simulink model "fly"  (Simulink 7.9)
settings: Solver=ode45  StartTime=0.0  StopTime=2  RelTol=1e-3
libraries: simulink x1
settings Model: Creator=tbourke  LastModifiedBy=tbourke

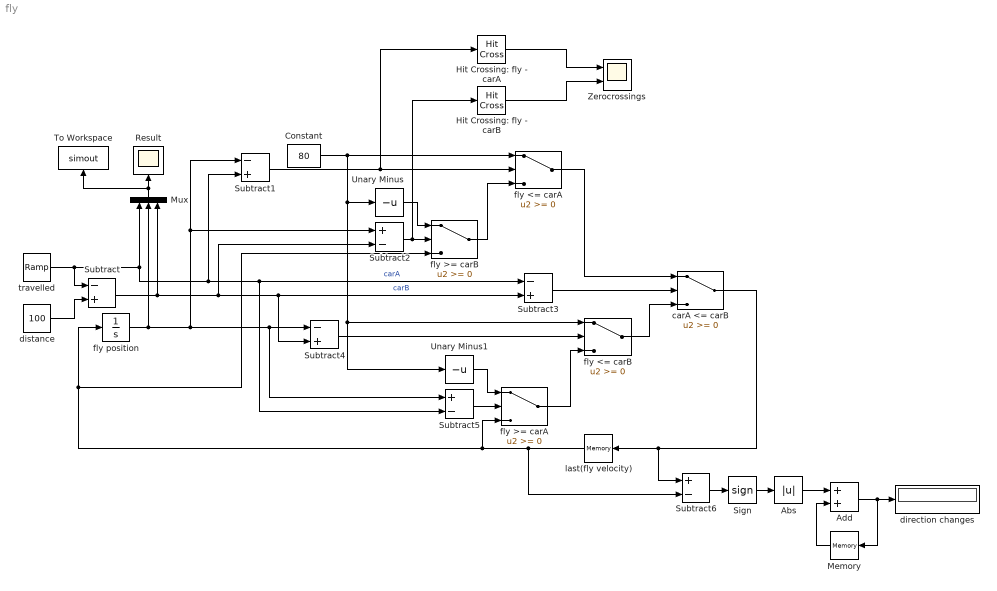
== system fly ==
  Abs : Abs
  Add : Sum
  Constant : Constant  Value=80
  Hit Crossing: fly - carA : HitCross
  Hit Crossing: fly - carB : HitCross
  Memory : Memory
  Mux : Mux  Inputs=3
  Result : Scope
      settings: TimeRange=2  YMin=0  YMax=100  SaveName=result  MaxDataPoints=500000  SampleInput=on
  Sign : Signum
  Subtract{,1,3..4} (4 alike) : Sum  Inputs=-+
  Subtract2 : Sum  Inputs=+-
  Subtract5 : Sum  Inputs=+-
  Subtract6 : Sum  Inputs=+-
  To Workspace : ToWorkspace  VariableName=simout  SampleTime=-1
  Unary Minus : UnaryMinus
  Unary Minus1 : UnaryMinus
  Zerocrossings : Scope  NumInputPorts=2
      settings: TimeRange=2  YMin=0~0  YMax=1~1  SaveName=zerocrossings  MaxDataPoints=500000  SampleInput=on
  carA <= carB : Switch
  direction changes : Display
  distance : Constant  Value=100
  fly <= carA : Switch
  fly <= carB : Switch
  fly >= carA : Switch
  fly >= carB : Switch
  fly position : Integrator
  last(fly velocity) : Memory  X0=80
  travelled : simulink/Sources/Ramp  slope=50  start=0  X0=0
  wires:
  Subtract3/1 -> carA <= carB/2
  distance/1 -> Subtract/2
  travelled/1 -> Subtract/1, Subtract1/2, Subtract3/1, Subtract5/2, Mux/1  "carA"
  Subtract/1 -> Subtract2/2, Subtract3/2, Subtract4/2, Mux/3  "carB"
  Subtract1/1 -> fly <= carA/2, Hit Crossing: fly - carA/1
  Subtract2/1 -> fly >= carB/2, Hit Crossing: fly - carB/1
  Constant/1 -> fly <= carA/1, Unary Minus/1, Unary Minus1/1, fly <= carB/1
  fly >= carB/1 -> fly <= carA/3
  Unary Minus/1 -> fly >= carB/1
  Subtract4/1 -> fly <= carB/2
  Subtract5/1 -> fly >= carA/2
  fly >= carA/1 -> fly <= carB/3
  Unary Minus1/1 -> fly >= carA/1
  last(fly velocity)/1 -> fly position/1, fly >= carB/3, fly >= carA/3, Subtract6/2
  fly position/1 -> Subtract1/1, Subtract2/1, Subtract4/1, Subtract5/1, Mux/2
  fly <= carA/1 -> carA <= carB/1
  carA <= carB/1 -> last(fly velocity)/1, Subtract6/1
  fly <= carB/1 -> carA <= carB/3
  Mux/1 -> To Workspace/1, Result/1
  Add/1 -> direction changes/1, Memory/1
  Memory/1 -> Add/2
  Subtract6/1 -> Sign/1
  Sign/1 -> Abs/1
  Abs/1 -> Add/1
  Hit Crossing: fly - carA/1 -> Zerocrossings/1
  Hit Crossing: fly - carB/1 -> Zerocrossings/2
